simulink model "Demo_MinSegNano"  (R2015a)
settings: Solver=FixedStepDiscrete  SolverMode=SingleTasking  StartTime=0.0  StopTime=inf  FixedStep=.03  RelTol=1e-3
PostLoadFcn:
  | try,
  | codertarget.arduinobase.registry.setBaudRate(gcs,115200)
  | disp('baud rate set to 115200 for external mode hardware serial')
  | baudrate='set_to_115200'
  | catch
  | disp('baud rate setting not needed in this version')
  | end
libraries: RASPlib x10, MinSegLibrary_MinSegNano x4, arduinolib x2
settings Model: ExtModeTrigDuration=2  Creator=Alec  LastModifiedBy=hurstj
settings OptimizationCC: ExpressionDepthLimit=2147483647  OptimizeModelRefInitCode=on  LifeSpan=1
settings DebuggingCC: UnderspecifiedInitializationDetection=Classic  MergeDetectMultiDrivingBlocksExec=none  StateNameClashWarn=warning
settings HardwareCC: ProdBitPerInt=16  ProdBitPerPointer=8  ProdIntDivRoundTo=Zero  ProdEndianess=LittleEndian  ProdWordSize=8  ProdHWDeviceType=Atmel->AVR
settings RTWCC: SystemTargetFile=realtime.tlc  GenerateMakefile=off  TemplateMakefile=realtime.tmf  Description=Real-Time Toolbox  RTWVerbose=off
settings CodeAppCC: CustomSymbolStrType=$N$R$M  InternalIdentifier=Classic
settings ERTTargetCC: CombineOutputUpdateFcns=off  ExtModeTransport=3  ExtModeMexArgs=0 1 9600  ERTSrcFileBannerTemplate=realtime_code_template.cgt  ERTHdrFileBannerTemplate=realtime_code_template.cgt  ERTDataSrcFileTemplate=realtime_code_template.cgt  ERTDataHdrFileTemplate=realtime_code_template.cgt  ERTCustomFileTemplate=realtime_file_process.tlc

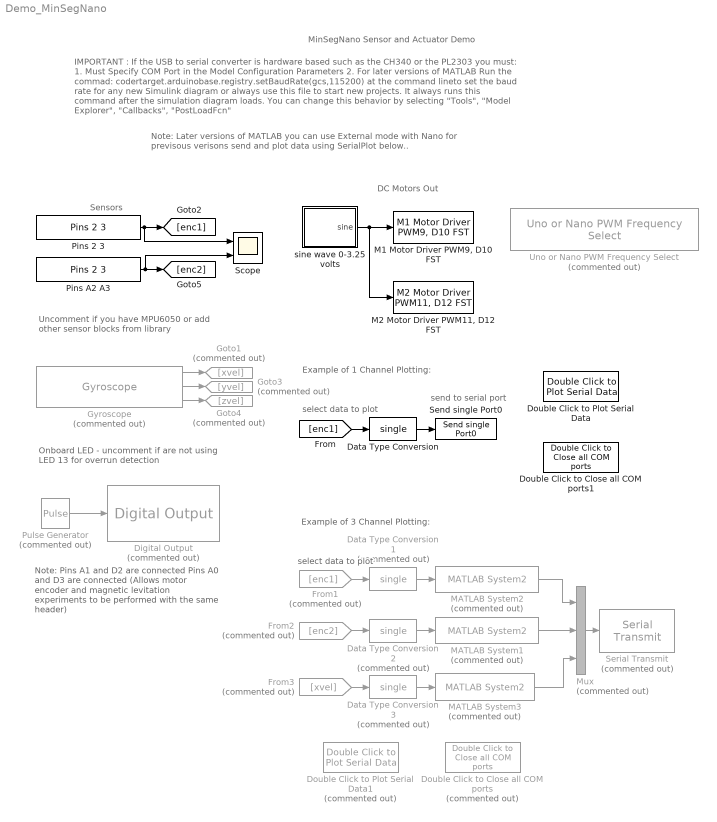
== system Demo_MinSegNano ==
  note: Note: Later versions of MATLAB you can use External mode with Nano
      |  for previsous verisons send and plot data using SerialPlot below..
  note: Onboard LED - uncomment if are not
      | using LED 13 for overrun detection
  note: Uncomment if you have MPU6050 or
      | add other sensor blocks from library
  note: Example of 1 Channel Plotting:
  note: send to serial port
  note: select data to plot
  note: DC Motors Out
  note: Sensors
  note: MinSegNano Sensor and Actuator Demo
  note: Example of 3 Channel Plotting:
  note: select data to plot
  note: IMPORTANT : If the USB to serial converter is hardware based such as the CH340 or the PL2303 you must:
      | 1. Must Specify COM Port in the Model Configuration Parameters
      | 2. For later versions of MATLAB Run the commad: codertarget.arduinobase.registry.setBaudRate(gcs,115200)
      | at the command lineto set the baud rate for any new Simulink diagram or always use this file to start new projects.
      | It always runs this command after the simulation diagram loads.
      | You can change this behavior by selecting "Tools", "Model Explorer", "Callbacks", "PostLoadFcn"
  note: Note: Pins  A1 and D2 are connected
      |          Pins  A0 and D3 are connected
      | (Allows  motor encoder and magnetic
      | levitation experiments to be performed
      | with the same header)
  Data Type Conversion : DataTypeConversion  OutDataTypeStr=single
  Data Type Conversion1 : DataTypeConversion  Commented=on  OutDataTypeStr=single
  Data Type Conversion2 : DataTypeConversion  Commented=on  OutDataTypeStr=single
  Data Type Conversion3 : DataTypeConversion  Commented=on  OutDataTypeStr=single
  Digital Output : arduinolib/Digital Output  Commented=on  pinNumber=13  blockPlatform=arduino
  Double Click to Close all COM ports : RASPlib/Double Click to Close all COM ports  Commented=on
  Double Click to Close all COM ports1 : RASPlib/Double Click to Close all COM ports
  Double Click to Plot Serial Data : RASPlib/Double Click to Plot Serial Data  COMport=89  BaudRate=9600  NumSamples=500  DataType=single  Ncx=1
  Double Click to Plot Serial Data1 : RASPlib/Double Click to Plot Serial Data  Commented=on  COMport=28  BaudRate=9600  NumSamples=500  DataType=single  Ncx=3
  From1 : From  Commented=on  GotoTag=enc1
  From2 : From  Commented=on  GotoTag=enc2
  From3 : From  Commented=on  GotoTag=xvel
  Goto1 : Goto  Commented=on  GotoTag=xvel
  Goto3 : Goto  Commented=on  GotoTag=yvel
  Goto4 : Goto  Commented=on  GotoTag=zvel
  Gyroscope : RASPlib/Gyroscope  Commented=on  DLPFmode=0
  "M1 Motor Driver PWM9, D10 FST" : MinSegLibrary_MinSegNano/M1 Motor Driver PWM9, D10 FST  Vsupply=3.25
  "M2 Motor Driver PWM11, D12 FST" : MinSegLibrary_MinSegNano/M2 Motor Driver PWM11, D12 FST  Vsupply=3.25
  MATLAB System1 : RASPlib/Send single Port0/MATLAB System2  Commented=on  SimulateUsing=Code generation
  MATLAB System2 : RASPlib/Send single Port0/MATLAB System2  Commented=on  SimulateUsing=Code generation
  MATLAB System3 : RASPlib/Send single Port0/MATLAB System2  Commented=on  SimulateUsing=Code generation
  Mux : Mux  Commented=on  Inputs=3
  Pins 2 3 : MinSegLibrary_MinSegNano/Pins 2 3  Encoder=0  PinA=2  PinB=3
  Pins A2 A3 : MinSegLibrary_MinSegNano/Pins 2 3  Encoder=4  PinA=16  PinB=17
  Pulse Generator : DiscretePulseGenerator  Commented=on  PulseType=Time based  Period=10  PulseWidth=5
  Scope : Scope  NumInputPorts=2
      settings: YMin=-5~-5  YMax=5~5
  Send single Port0 : RASPlib/Send single Port0
  Serial Transmit : arduinolib/Serial Transmit  Commented=on  portNumber=0  blockPlatform=arduino
  Uno or Nano PWM Frequency Select : RASPlib/Uno or Nano PWM Frequency Select  Commented=on  Frequency=490Hz (Timer 0: 976Hz)  Timer=1 - pins 9, 10
  sine wave 0-3.25 volts : Subsystem
  wires:
  Pins 2 3/1 -> Scope/1, [enc1]
  [enc1] -> Data Type Conversion/1
  Data Type Conversion/1 -> Send single Port0/1
  Gyroscope/1 -> Goto1/1
  MATLAB System1/1 -> Mux/2
  MATLAB System2/1 -> Mux/1
  From1/1 -> Data Type Conversion1/1
  Data Type Conversion1/1 -> MATLAB System2/1
  From2/1 -> Data Type Conversion2/1
  Data Type Conversion2/1 -> MATLAB System1/1
  Mux/1 -> Serial Transmit/1
  Data Type Conversion3/1 -> MATLAB System3/1
  MATLAB System3/1 -> Mux/3
  From3/1 -> Data Type Conversion3/1
  Pulse Generator/1 -> Digital Output/1
  Gyroscope/2 -> Goto3/1
  Gyroscope/3 -> Goto4/1
  sine wave 0-3.25 volts/1(sine) -> "M2 Motor Driver PWM11, D12 FST"/1, "M1 Motor Driver PWM9, D10 FST"/1
  Pins A2 A3/1 -> Scope/2, [enc2]

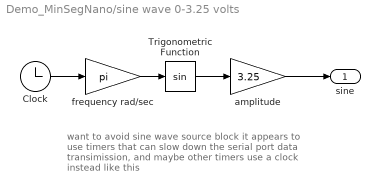
== system Demo_MinSegNano/sine wave 0-3.25 volts ==
  note: want to avoid sine wave source block
      | it appears to use timers that can slow down the
      | serial port data transimission, and maybe
      | other timers
      |
      | use a clock instead like this
  Clock : Clock
  Trigonometric Function : Trigonometry
  amplitude : Gain  Gain=3.25
  frequency rad/sec : Gain  Gain=pi
  sine : Outport
  wires:
  Clock/1 -> frequency rad/sec/1
  Trigonometric Function/1 -> amplitude/1
  frequency rad/sec/1 -> Trigonometric Function/1
  amplitude/1 -> sine/1
